simulink model "part3and4"  (R2021b)
settings: Solver=ode23s  StartTime=0.0  StopTime=100  RelTol=1e-3
settings Model: Creator=User  LastModifiedBy=User

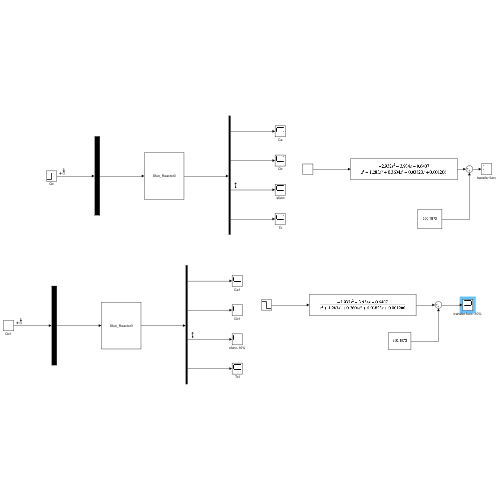
[thumbnail: Simulink's stored preview of the top-level diagram]
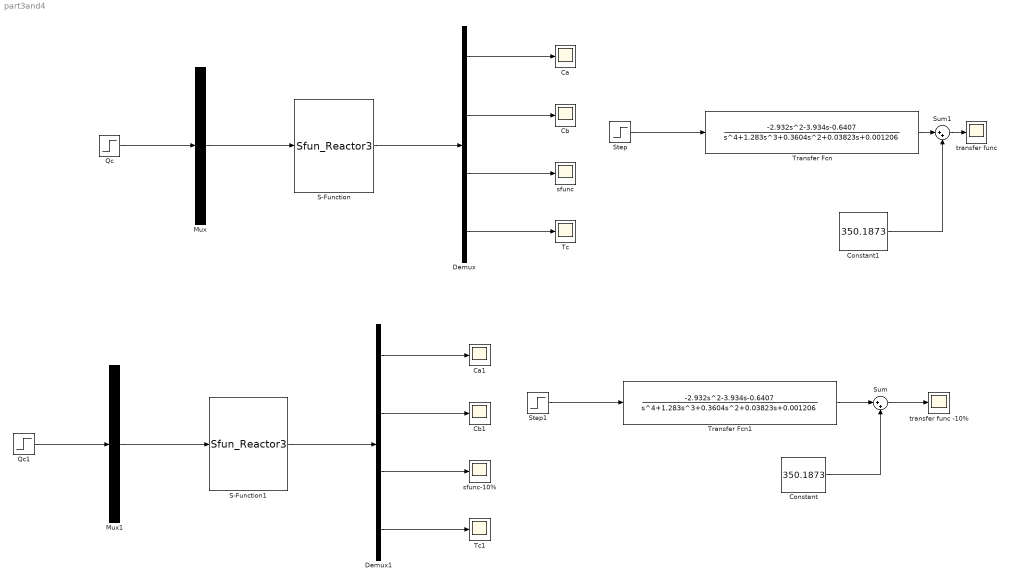
== system part3and4 ==
  " Tc" : Scope
  " Tc1" : Scope
  " sfunc" : Scope
  Ca : Scope
  Ca1 : Scope
  Cb : Scope
  Cb1 : Scope
  Constant : Constant  Value=350.1873
  Constant1 : Constant  Value=350.1873
  Demux : Demux
  Demux1 : Demux
  Mux : Mux  Inputs=1
  Mux1 : Mux  Inputs=1
  Qc : Step  Time=5  Before=0.03  After=0.033  SampleTime=0
  Qc1 : Step  Time=5  Before=0.03  After=0.027  SampleTime=0
  S-Function : S-Function  FunctionName=Sfun_Reactor3  SFunctionDeploymentMode=off  EnableBusSupport=off
  S-Function1 : S-Function  FunctionName=Sfun_Reactor3  SFunctionDeploymentMode=off  EnableBusSupport=off
  Step : Step  Time=5  After=0.003  SampleTime=0
  Step1 : Step  Time=5  After=-0.003  SampleTime=0
  Sum : Sum  Inputs=|++
  Sum1 : Sum  Inputs=|++
  Transfer Fcn : TransferFcn  Numerator=[-2.932 -3.934 -0.6407]  Denominator=[1 1.283 0.3604 0.03823 0.001206]
  Transfer Fcn1 : TransferFcn  Numerator=[-2.932 -3.934 -0.6407]  Denominator=[1 1.283 0.3604 0.03823 0.001206]
  sfunc-10% : Scope
  transfer func : Scope
  transfer func -10% : Scope
  wires:
  Mux/1 -> S-Function/1
  S-Function/1 -> Demux/1
  Demux/2 -> Cb/1
  Demux/3 -> " sfunc"/1
  Demux/4 -> " Tc"/1
  Demux/1 -> Ca/1
  Qc/1 -> Mux/1
  Step/1 -> Transfer Fcn/1
  Qc1/1 -> Mux1/1
  Demux1/1 -> Ca1/1
  Demux1/4 -> " Tc1"/1
  Demux1/3 -> sfunc-10%/1
  Demux1/2 -> Cb1/1
  S-Function1/1 -> Demux1/1
  Mux1/1 -> S-Function1/1
  Step1/1 -> Transfer Fcn1/1
  Constant1/1 -> Sum1/2
  Transfer Fcn/1 -> Sum1/1
  Sum1/1 -> transfer func/1
  Constant/1 -> Sum/2
  Transfer Fcn1/1 -> Sum/1
  Sum/1 -> transfer func -10%/1
